simulink model "model"  (R2024a)
settings: Solver=VariableStepAuto  StartTime=0.0  StopTime=30  FixedStep=0.000001  RelTol=1e-10  AbsTol=1e-10
values from neighbouring files (symbols this model uses):
  A = [1, 0 ... (first row only)    [calc.m]    (also in prep.m = [1 0; 0 0])
  A0f = [0    1 ... (first row only)    [calc.m]    (also in prep.m = [0 1; -0.25 -1])
  b = [2 ... (first row only)    [calc.m]    (also in prep.m = [2; 4])
  d = [2 ... (first row only)    [calc.m]    (also in prep.m = [2; 4])
  K = H * inv(M)    [calc.m]    (also in prep.m)
  N = b0f/d    [calc.m]    (also in prep.m)
  P = lyap(Am', Q)    [prep.m]
settings Model: Creator=ventus  LastModifiedBy=ventus
settings OptimizationCC: EnhancedBackFolding=on  PassReuseOutputArgsAs=Individual arguments  ZeroExternalMemoryAtStartup=off  ZeroInternalMemoryAtStartup=off  MaxStackSize=64  OptimizeBlockOrder=speed  DifferentSizesBufferReuse=on  OptimizationCustomize=off  EfficientTunableParamExpr=on
settings DebuggingCC: ParameterTunabilityLossMsg=error
settings SFSimCC: MATLABDynamicMemAlloc=off
settings RTWCC: Description=Embedded Coder  SystemTargetFile=ert.tlc  HardwareBoard=Robot Operating System 2 (ROS 2)  TLCOptions="-aInlineSetEventsForThisBaseRateFcn=TLC_FALSE -aSuppressMultiTaskScheduler=TLC_FALSE  -aRateBasedStepFcn=0"  TemplateMakefile=ert_default_tmf  Toolchain=Colcon Tools  TargetLang=C++
settings CodeAppCC: ForceParamTrailComments=on  IgnoreCustomStorageClasses=off  OperatorAnnotations=on  SimulinkDataObjDesc=on  SFDataObjDesc=on  InsertBlockDesc=on
settings ERTTargetCC: CodeInterfacePackaging=C++ class  RootIOFormat=Structure reference

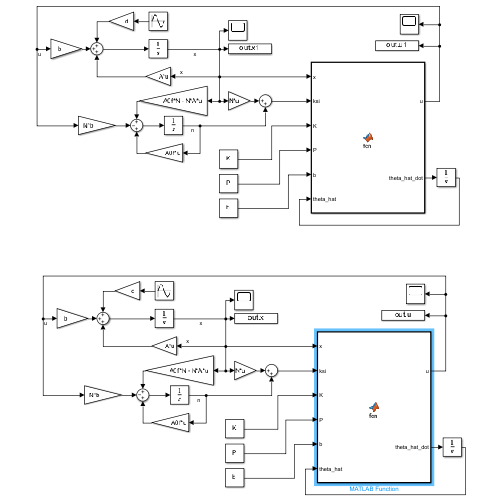
[thumbnail: Simulink's stored preview of the top-level diagram]
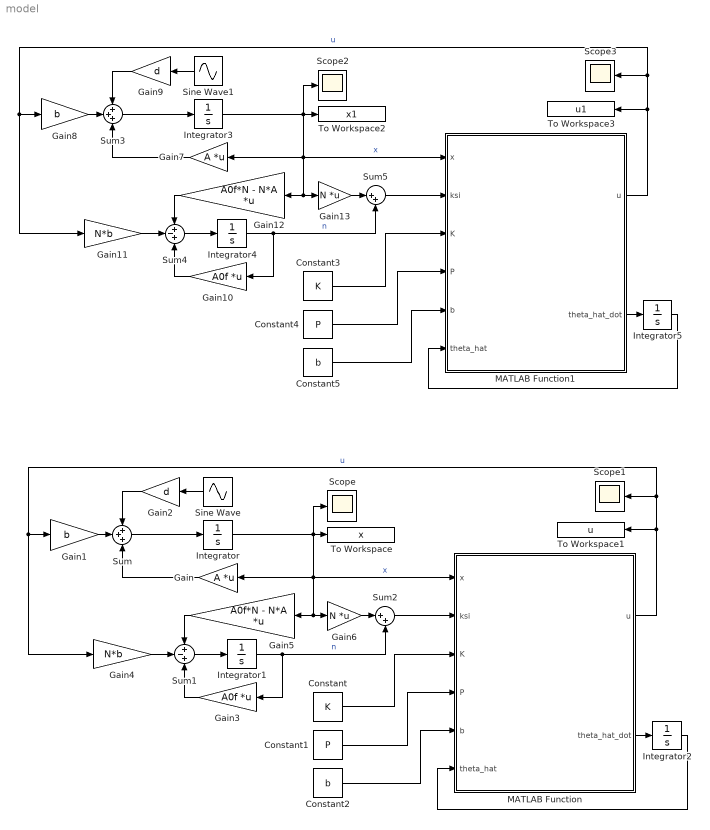
== system model ==
  Constant : Constant  Value=K  VectorParams1D=off
  Constant1 : Constant  Value=P  VectorParams1D=off
  Constant2 : Constant  Value=b  VectorParams1D=off
  Constant3 : Constant  Value=K  VectorParams1D=off
  Constant4 : Constant  Value=P  VectorParams1D=off
  Constant5 : Constant  Value=b  VectorParams1D=off
  Gain : Gain  Gain=A  Multiplication=Matrix(K*u)
  Gain1 : Gain  Gain=b
  Gain10 : Gain  Gain=A0f  Multiplication=Matrix(K*u)
  Gain11 : Gain  Gain=N*b
  Gain12 : Gain  Gain=A0f*N - N*A  Multiplication=Matrix(K*u)
  Gain13 : Gain  Gain=N  Multiplication=Matrix(K*u)
  Gain2 : Gain  Gain=d
  Gain3 : Gain  Gain=A0f  Multiplication=Matrix(K*u)
  Gain4 : Gain  Gain=N*b
  Gain5 : Gain  Gain=A0f*N - N*A  Multiplication=Matrix(K*u)
  Gain6 : Gain  Gain=N  Multiplication=Matrix(K*u)
  Gain7 : Gain  Gain=A  Multiplication=Matrix(K*u)
  Gain8 : Gain  Gain=b
  Gain9 : Gain  Gain=d
  Integrator{,1..5} (6 alike) : Integrator  InitialCondition=[0; 0]
  MATLAB Function : MATLAB Function  TreatAsAtomicUnit=on
  MATLAB Function1 : MATLAB Function  TreatAsAtomicUnit=on
  Scope{,1..3} (4 alike) : Scope
  Sine Wave : Sin  Amplitude=2  SampleTime=0
  Sine Wave1 : Sin  Amplitude=2  SampleTime=0
  Sum : Sum  Inputs=+++
  Sum1 : Sum  Inputs=+-+
  Sum2 : Sum  Inputs=|++
  Sum3 : Sum  Inputs=+++
  Sum4 : Sum  Inputs=+-+
  Sum5 : Sum  Inputs=|++
  To Workspace : ToWorkspace  VariableName=x  SaveFormat=Timeseries  SampleTime=-1
  To Workspace1 : ToWorkspace  VariableName=u  SaveFormat=Timeseries  SampleTime=-1
  To Workspace2 : ToWorkspace  VariableName=x1  SaveFormat=Timeseries  SampleTime=-1
  To Workspace3 : ToWorkspace  VariableName=u1  SaveFormat=Timeseries  SampleTime=-1
  wires:
  Sum/1 -> Integrator/1
  Integrator/1 -> To Workspace/1, Gain/1, Gain5/1, Gain6/1, MATLAB Function/1(x), Scope/1  "x"
  Gain/1 -> Sum/3
  Gain2/1 -> Sum/1
  Sine Wave/1 -> Gain2/1
  Sum1/1 -> Integrator1/1
  Integrator1/1 -> Gain3/1, Sum2/2  "n"
  Gain3/1 -> Sum1/3
  Gain4/1 -> Sum1/2
  Gain5/1 -> Sum1/1
  Gain6/1 -> Sum2/1
  Sum2/1 -> MATLAB Function/2(ksi)
  MATLAB Function/2(theta_hat_dot) -> Integrator2/1
  Integrator2/1 -> MATLAB Function/6(theta_hat)
  MATLAB Function/1(u) -> To Workspace1/1, Scope1/1, Gain1/1, Gain4/1  "u"
  Constant/1 -> MATLAB Function/3(K)
  Constant1/1 -> MATLAB Function/4(P)
  Constant2/1 -> MATLAB Function/5(b)
  Gain1/1 -> Sum/2
  Gain9/1 -> Sum3/1
  Gain8/1 -> Sum3/2
  Constant4/1 -> MATLAB Function1/4(P)
  Constant5/1 -> MATLAB Function1/5(b)
  MATLAB Function1/1(u) -> To Workspace3/1, Scope3/1, Gain8/1, Gain11/1  "u"
  Constant3/1 -> MATLAB Function1/3(K)
  Gain12/1 -> Sum4/1
  Sine Wave1/1 -> Gain9/1
  Gain13/1 -> Sum5/1
  MATLAB Function1/2(theta_hat_dot) -> Integrator5/1
  Gain11/1 -> Sum4/2
  Gain10/1 -> Sum4/3
  Integrator3/1 -> To Workspace2/1, Gain7/1, Gain12/1, Gain13/1, MATLAB Function1/1(x), Scope2/1  "x"
  Integrator4/1 -> Gain10/1, Sum5/2  "n"
  Gain7/1 -> Sum3/3
  Sum5/1 -> MATLAB Function1/2(ksi)
  Integrator5/1 -> MATLAB Function1/6(theta_hat)
  Sum4/1 -> Integrator4/1
  Sum3/1 -> Integrator3/1

== matlab function model/MATLAB Function1 ==
  data: u output; x input; ksi input; K input; P input; b input; theta_hat input; theta_hat_dot output
function [u, theta_hat_dot] = fcn(x, ksi, K, P, b, theta_hat)
gamma = 100;
u = -K*x -theta_hat'*ksi;

theta_hat_dot = gamma*ksi*b'*P*x;

== matlab function model/MATLAB Function ==
  data: u output; x input; ksi input; K input; P input; b input; theta_hat input; theta_hat_dot output
function [u, theta_hat_dot] = fcn(x, ksi, K, P, b, theta_hat)
gamma = 10;
u = -K*x -theta_hat'*ksi;

theta_hat_dot = gamma*ksi*b'*P*x;
